simulink model "kundur_cvs_v3"  (R2025b)
settings: Solver=ode23t  StartTime=0.0  StopTime=0.5  MaxStep=0.005  RelTol=1e-3
values from neighbouring files (symbols this model uses):
  CCS_Load_amp_bus7 = 0    [kundur_cvs_v3_discrete_runtime.mat]    (also in kundur_cvs_v3_runtime.mat)
  CCS_Load_amp_bus9 = 0    [kundur_cvs_v3_discrete_runtime.mat]    (also in kundur_cvs_v3_runtime.mat)
  delta0_1 = 0.294539737007    [kundur_cvs_v3_discrete_runtime.mat]    (also in kundur_cvs_v3_runtime.mat)
  delta0_2 = 0.0944024626245    [kundur_cvs_v3_discrete_runtime.mat]    (also in kundur_cvs_v3_runtime.mat)
  delta0_3 = 0.25103283995    [kundur_cvs_v3_discrete_runtime.mat]    (also in kundur_cvs_v3_runtime.mat)
  delta0_4 = 0.0812572055811    [kundur_cvs_v3_discrete_runtime.mat]    (also in kundur_cvs_v3_runtime.mat)
  deltaG0_1 = 0.522124293082    [kundur_cvs_v3_discrete_runtime.mat]    (also in kundur_cvs_v3_runtime.mat)
  deltaG0_2 = 0.476153951225    [kundur_cvs_v3_discrete_runtime.mat]    (also in kundur_cvs_v3_runtime.mat)
  deltaG0_3 = 0.293879837027    [kundur_cvs_v3_discrete_runtime.mat]    (also in kundur_cvs_v3_runtime.mat)
  Dg_1 = 5    [kundur_cvs_v3_discrete_runtime.mat]    (also in kundur_cvs_v3_runtime.mat)
  Dg_2 = 5    [kundur_cvs_v3_discrete_runtime.mat]    (also in kundur_cvs_v3_runtime.mat)
  Dg_3 = 5    [kundur_cvs_v3_discrete_runtime.mat]    (also in kundur_cvs_v3_runtime.mat)
  LoadStep_amp_bus14 = 248000000    [kundur_cvs_v3_discrete_runtime.mat]    (also in kundur_cvs_v3_runtime.mat)
  LoadStep_amp_bus15 = 0    [kundur_cvs_v3_discrete_runtime.mat]    (also in kundur_cvs_v3_runtime.mat)
  LoadStep_trip_amp_bus14 = 0    [kundur_cvs_v3_discrete_runtime.mat]    (also in kundur_cvs_v3_runtime.mat)
  LoadStep_trip_amp_bus15 = 0    [kundur_cvs_v3_discrete_runtime.mat]    (also in kundur_cvs_v3_runtime.mat)
  Mg_1 = 13    [kundur_cvs_v3_discrete_runtime.mat]    (also in kundur_cvs_v3_runtime.mat)
  Mg_2 = 13    [kundur_cvs_v3_discrete_runtime.mat]    (also in kundur_cvs_v3_runtime.mat)
  Mg_3 = 12.35    [kundur_cvs_v3_discrete_runtime.mat]    (also in kundur_cvs_v3_runtime.mat)
  Pe_scale = 1e-08    [kundur_cvs_runtime.mat]    (also in kundur_cvs_v3_discrete_runtime.mat; kundur_cvs_v3_runtime.mat)
  Pm_1 = 0.250224865012    [kundur_cvs_v3_discrete_runtime.mat]    (also in kundur_cvs_v3_runtime.mat)
  Pm_2 = 0.250224865012    [kundur_cvs_v3_discrete_runtime.mat]    (also in kundur_cvs_v3_runtime.mat)
  Pm_3 = 0.250224865012    [kundur_cvs_v3_discrete_runtime.mat]    (also in kundur_cvs_v3_runtime.mat)
  Pm_4 = 0.250224865012    [kundur_cvs_v3_discrete_runtime.mat]    (also in kundur_cvs_v3_runtime.mat)
  Pmg_1 = 7.00000000011    [kundur_cvs_v3_discrete_runtime.mat]    (also in kundur_cvs_v3_runtime.mat)
  Pmg_2 = 7    [kundur_cvs_v3_discrete_runtime.mat]    (also in kundur_cvs_v3_runtime.mat)
  Pmg_3 = 7.19    [kundur_cvs_v3_discrete_runtime.mat]    (also in kundur_cvs_v3_runtime.mat)
  PmgStep_amp_1 = 0    [kundur_cvs_v3_discrete_runtime.mat]    (also in kundur_cvs_v3_runtime.mat)
  PmgStep_amp_2 = 0    [kundur_cvs_v3_discrete_runtime.mat]    (also in kundur_cvs_v3_runtime.mat)
  PmgStep_amp_3 = 0    [kundur_cvs_v3_discrete_runtime.mat]    (also in kundur_cvs_v3_runtime.mat)
  PmgStep_t_1 = 5    [kundur_cvs_v3_discrete_runtime.mat]    (also in kundur_cvs_v3_runtime.mat)
  PmgStep_t_2 = 5    [kundur_cvs_v3_discrete_runtime.mat]    (also in kundur_cvs_v3_runtime.mat)
  PmgStep_t_3 = 5    [kundur_cvs_v3_discrete_runtime.mat]    (also in kundur_cvs_v3_runtime.mat)
  Rg_1 = 0.05    [kundur_cvs_v3_discrete_runtime.mat]    (also in kundur_cvs_v3_runtime.mat)
  Rg_2 = 0.05    [kundur_cvs_v3_discrete_runtime.mat]    (also in kundur_cvs_v3_runtime.mat)
  Rg_3 = 0.05    [kundur_cvs_v3_discrete_runtime.mat]    (also in kundur_cvs_v3_runtime.mat)
  SGScale_1 = 0.111111111111    [kundur_cvs_v3_discrete_runtime.mat]    (also in kundur_cvs_v3_runtime.mat)
  SGScale_2 = 0.111111111111    [kundur_cvs_v3_discrete_runtime.mat]    (also in kundur_cvs_v3_runtime.mat)
  SGScale_3 = 0.111111111111    [kundur_cvs_v3_discrete_runtime.mat]    (also in kundur_cvs_v3_runtime.mat)
  Vbase_const = 230000    [kundur_cvs_runtime.mat]    (also in kundur_cvs_v3_discrete_runtime.mat; kundur_cvs_v3_runtime.mat)
  VemfG_1 = 266775.927939    [kundur_cvs_v3_discrete_runtime.mat]    (also in kundur_cvs_v3_runtime.mat)
  VemfG_2 = 255963.649879    [kundur_cvs_v3_discrete_runtime.mat]    (also in kundur_cvs_v3_runtime.mat)
  VemfG_3 = 266432.593136    [kundur_cvs_v3_discrete_runtime.mat]    (also in kundur_cvs_v3_runtime.mat)
  Vmag_1 = 230000    [kundur_cvs_runtime.mat]    (also in kundur_cvs_v3_discrete_runtime.mat = 201813.659575; kundur_cvs_v3_runtime.mat = 201813.659575)
  Vmag_2 = 230000    [kundur_cvs_runtime.mat]    (also in kundur_cvs_v3_discrete_runtime.mat = 232642.850172; kundur_cvs_v3_runtime.mat = 232642.850172)
  Vmag_3 = 230000    [kundur_cvs_runtime.mat]    (also in kundur_cvs_v3_discrete_runtime.mat = 178957.562058; kundur_cvs_v3_runtime.mat = 178957.562058)
  Vmag_4 = 230000    [kundur_cvs_runtime.mat]    (also in kundur_cvs_v3_discrete_runtime.mat = 226974.072481; kundur_cvs_v3_runtime.mat = 226974.072481)
  VSGScale_1 = 0.5    [kundur_cvs_v3_discrete_runtime.mat]    (also in kundur_cvs_v3_runtime.mat)
  VSGScale_2 = 0.5    [kundur_cvs_v3_discrete_runtime.mat]    (also in kundur_cvs_v3_runtime.mat)
  VSGScale_3 = 0.5    [kundur_cvs_v3_discrete_runtime.mat]    (also in kundur_cvs_v3_runtime.mat)
  VSGScale_4 = 0.5    [kundur_cvs_v3_discrete_runtime.mat]    (also in kundur_cvs_v3_runtime.mat)
  WindAmp_1 = 1    [kundur_cvs_v3_discrete_runtime.mat]    (also in kundur_cvs_v3_runtime.mat)
  WindAmp_2 = 1    [kundur_cvs_v3_discrete_runtime.mat]    (also in kundur_cvs_v3_runtime.mat)
  wn_const = 314.159265359    [kundur_cvs_runtime.mat]    (also in kundur_cvs_v3_discrete_runtime.mat; kundur_cvs_v3_runtime.mat)
  Wphase_1 = 0.0648179941055    [kundur_cvs_v3_discrete_runtime.mat]    (also in kundur_cvs_v3_runtime.mat)
  Wphase_2 = 0.0587091014116    [kundur_cvs_v3_discrete_runtime.mat]    (also in kundur_cvs_v3_runtime.mat)
  WVmag_1 = 230000    [kundur_cvs_v3_discrete_runtime.mat]    (also in kundur_cvs_v3_runtime.mat)
  WVmag_2 = 230000    [kundur_cvs_v3_discrete_runtime.mat]    (also in kundur_cvs_v3_runtime.mat)
undefined symbols (not defined in the file or in its folder): D_1, D_2, D_3, D_4, M_1, M_2, M_3, M_4, Pm_step_amp_1, Pm_step_amp_2, Pm_step_amp_3, Pm_step_amp_4, Pm_step_t_1, Pm_step_t_2, Pm_step_t_3, Pm_step_t_4
libraries: spsSeriesRLCBranchLib x72, spsGroundLib x57, spsControlledVoltageSourceLib x7, spsCurrentMeasurementLib x7, spsVoltageMeasurementLib x7, spsControlledCurrentSourceLib x4, spsACVoltageSourceLib x2, spspowerguiLib x1
settings Model: Creator=27443  LastModifiedBy=27443

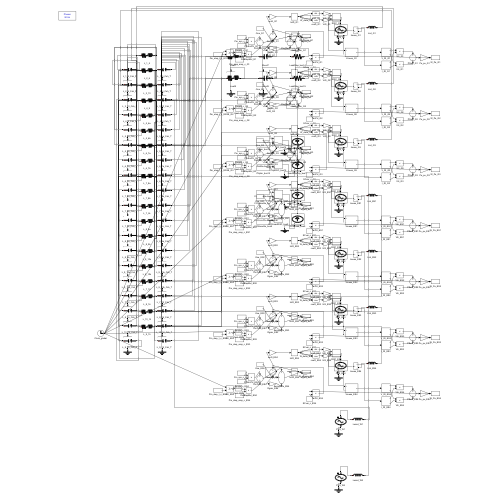
[thumbnail: Simulink's stored preview of the top-level diagram]
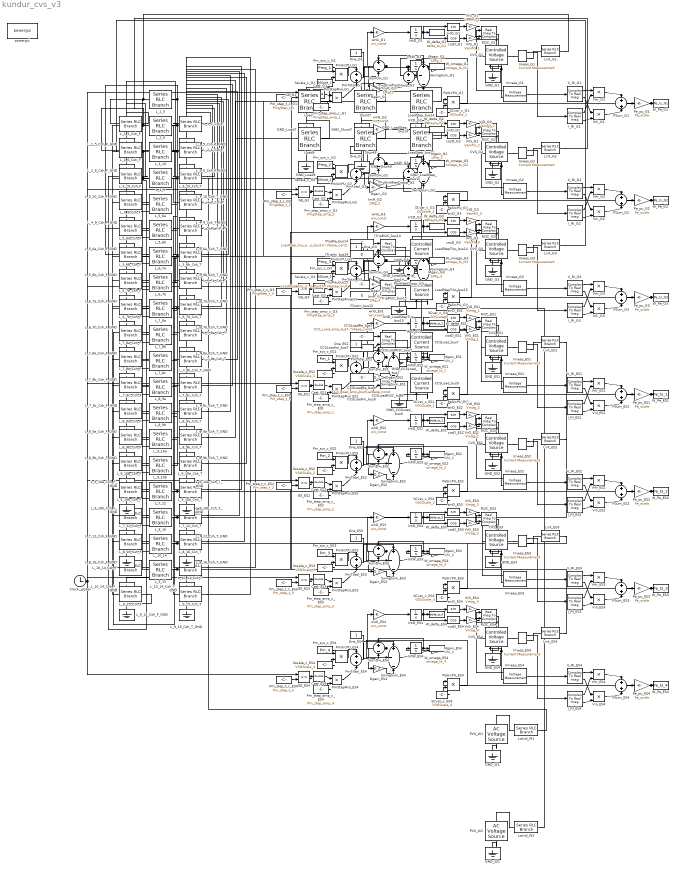
== system kundur_cvs_v3 ==
  CCSLoadIm_bus7 : Constant  Value=0
  CCSLoadIm_bus9 : Constant  Value=0
  CCSLoadRI2C_bus7 : RealImagToComplex
  CCSLoadRI2C_bus9 : RealImagToComplex
  CCSLoadRe_bus7 : Constant  Value=CCS_Load_amp_bus7 / Vbase_const
  CCSLoadRe_bus9 : Constant  Value=CCS_Load_amp_bus9 / Vbase_const
  CCSLoad_bus7 : spsControlledCurrentSourceLib/Controlled Current Source  Initialize=off  Source_Type=AC  Amplitude=0  Phase=0  Frequency=0  Measurements=None
  CCSLoad_bus9 : spsControlledCurrentSourceLib/Controlled Current Source  Initialize=off  Source_Type=AC  Amplitude=0  Phase=0  Frequency=0  Measurements=None
  CVS_ES1 : spsControlledVoltageSourceLib/Controlled Voltage Source  Initialize=off  Source_Type=DC  Amplitude=Vmag_1  Phase=0  Frequency=0  Measurements=None
  CVS_ES2 : spsControlledVoltageSourceLib/Controlled Voltage Source  Initialize=off  Source_Type=DC  Amplitude=Vmag_2  Phase=0  Frequency=0  Measurements=None
  CVS_ES3 : spsControlledVoltageSourceLib/Controlled Voltage Source  Initialize=off  Source_Type=DC  Amplitude=Vmag_3  Phase=0  Frequency=0  Measurements=None
  CVS_ES4 : spsControlledVoltageSourceLib/Controlled Voltage Source  Initialize=off  Source_Type=DC  Amplitude=Vmag_4  Phase=0  Frequency=0  Measurements=None
  CVS_G1 : spsControlledVoltageSourceLib/Controlled Voltage Source  Initialize=off  Source_Type=DC  Amplitude=VemfG_1  Phase=0  Frequency=0  Measurements=None
  CVS_G2 : spsControlledVoltageSourceLib/Controlled Voltage Source  Initialize=off  Source_Type=DC  Amplitude=VemfG_2  Phase=0  Frequency=0  Measurements=None
  CVS_G3 : spsControlledVoltageSourceLib/Controlled Voltage Source  Initialize=off  Source_Type=DC  Amplitude=VemfG_3  Phase=0  Frequency=0  Measurements=None
  Cast_ES{1..4} (4 alike) : DataTypeConversion  OutDataTypeStr=double  SaturateOnIntegerOverflow=off  RndMeth=Floor
  Cast_G1 : DataTypeConversion  OutDataTypeStr=double  SaturateOnIntegerOverflow=off  RndMeth=Floor
  Cast_G2 : DataTypeConversion  OutDataTypeStr=double  SaturateOnIntegerOverflow=off  RndMeth=Floor
  Cast_G3 : DataTypeConversion  OutDataTypeStr=double  SaturateOnIntegerOverflow=off  RndMeth=Floor
  Clock_global : Clock
  Dgain_ES1 : Gain  Gain=D_1
  Dgain_ES2 : Gain  Gain=D_2
  Dgain_ES3 : Gain  Gain=D_3
  Dgain_ES4 : Gain  Gain=D_4
  Dgain_G1 : Gain  Gain=Dg_1
  Dgain_G2 : Gain  Gain=Dg_2
  Dgain_G3 : Gain  Gain=Dg_3
  GE_ES{1..4} (4 alike) : RelationalOperator  OutDataTypeStr=boolean  RndMeth=Simplest  InputSameDT=off
  GE_G1 : RelationalOperator  OutDataTypeStr=boolean  RndMeth=Simplest  InputSameDT=off
  GE_G2 : RelationalOperator  OutDataTypeStr=boolean  RndMeth=Simplest  InputSameDT=off
  GE_G3 : RelationalOperator  OutDataTypeStr=boolean  RndMeth=Simplest  InputSameDT=off
  GND_CCSLoad_bus7 : spsGroundLib/Ground  LConnTagsString=a
  GND_CCSLoad_bus9 : spsGroundLib/Ground  LConnTagsString=a
  GND_ES{1..4} (4 alike) : spsGroundLib/Ground  LConnTagsString=a
  GND_G1 : spsGroundLib/Ground  LConnTagsString=a
  GND_G2 : spsGroundLib/Ground  LConnTagsString=a
  GND_G3 : spsGroundLib/Ground  LConnTagsString=a
  GND_Load7 : spsGroundLib/Ground  LConnTagsString=a
  GND_Load9 : spsGroundLib/Ground  LConnTagsString=a
  GND_LoadStepTrip_bus14 : spsGroundLib/Ground  LConnTagsString=a
  GND_LoadStepTrip_bus15 : spsGroundLib/Ground  LConnTagsString=a
  GND_LoadStep_bus14 : spsGroundLib/Ground  LConnTagsString=a
  GND_LoadStep_bus15 : spsGroundLib/Ground  LConnTagsString=a
  GND_Shunt7 : spsGroundLib/Ground  LConnTagsString=a
  GND_Shunt9 : spsGroundLib/Ground  LConnTagsString=a
  GND_W1 : spsGroundLib/Ground  LConnTagsString=a
  GND_W2 : spsGroundLib/Ground  LConnTagsString=a
  ITripIm_bus14 : Constant  Value=0
  ITripIm_bus15 : Constant  Value=0
  ITripRI2C_bus14 : RealImagToComplex
  ITripRI2C_bus15 : RealImagToComplex
  ITripRe_bus14 : Constant  Value=LoadStep_trip_amp_bus14 / Vbase_const
  ITripRe_bus15 : Constant  Value=LoadStep_trip_amp_bus15 / Vbase_const
  I_RI_ES{1..4} (4 alike) : ComplexToRealImag
  I_RI_G1 : ComplexToRealImag
  I_RI_G2 : ComplexToRealImag
  I_RI_G3 : ComplexToRealImag
  Imeas_ES{1..4} (4 alike) : spsCurrentMeasurementLib/Current Measurement  PhasorSimulation=on  OutputType=Complex  PSBequivalent=0
  Imeas_G1 : spsCurrentMeasurementLib/Current Measurement  PhasorSimulation=on  OutputType=Complex  PSBequivalent=0
  Imeas_G2 : spsCurrentMeasurementLib/Current Measurement  PhasorSimulation=on  OutputType=Complex  PSBequivalent=0
  Imeas_G3 : spsCurrentMeasurementLib/Current Measurement  PhasorSimulation=on  OutputType=Complex  PSBequivalent=0
  IntD_ES1 : Integrator  InitialCondition=delta0_1
  IntD_ES2 : Integrator  InitialCondition=delta0_2
  IntD_ES3 : Integrator  InitialCondition=delta0_3
  IntD_ES4 : Integrator  InitialCondition=delta0_4
  IntD_G1 : Integrator  InitialCondition=deltaG0_1
  IntD_G2 : Integrator  InitialCondition=deltaG0_2
  IntD_G3 : Integrator  InitialCondition=deltaG0_3
  IntW_ES{1..4} (4 alike) : Integrator  InitialCondition=1
  IntW_G1 : Integrator  InitialCondition=1
  IntW_G2 : Integrator  InitialCondition=1
  IntW_G3 : Integrator  InitialCondition=1
  InvR_G1 : Gain  Gain=1/Rg_1
  InvR_G2 : Gain  Gain=1/Rg_2
  InvR_G3 : Gain  Gain=1/Rg_3
  L_10_14 : spsSeriesRLCBranchLib/Series RLC Branch  LConnTagsString=__new0  RConnTagsString=__new0  BranchType=RL  Resistance=0.01  Inductance=0.0005  SetiL0=off  InitialCurrent=0  Capacitance=1e-6  Setx0=off  InitialVoltage=0  Measurements=None
  L_10_14_Csh_F : spsSeriesRLCBranchLib/Series RLC Branch  LConnTagsString=__new0  RConnTagsString=__new0  BranchType=C  Resistance=1  Inductance=1e-3  SetiL0=off  InitialCurrent=0  Capacitance=4.5e-09  Setx0=off  InitialVoltage=0  Measurements=None
  L_10_14_Csh_F_GND : spsGroundLib/Ground  LConnTagsString=a
  L_10_14_Csh_T : spsSeriesRLCBranchLib/Series RLC Branch  LConnTagsString=__new0  RConnTagsString=__new0  BranchType=C  Resistance=1  Inductance=1e-3  SetiL0=off  InitialCurrent=0  Capacitance=4.5e-09  Setx0=off  InitialVoltage=0  Measurements=None
  L_10_14_Csh_T_GND : spsGroundLib/Ground  LConnTagsString=a
  L_1_5 : spsSeriesRLCBranchLib/Series RLC Branch  LConnTagsString=__new0  RConnTagsString=__new0  BranchType=RL  Resistance=0.265  Inductance=0.00705  SetiL0=off  InitialCurrent=0  Capacitance=1e-6  Setx0=off  InitialVoltage=0  Measurements=None
  L_1_5_Csh_F : spsSeriesRLCBranchLib/Series RLC Branch  LConnTagsString=__new0  RConnTagsString=__new0  BranchType=C  Resistance=1  Inductance=1e-3  SetiL0=off  InitialCurrent=0  Capacitance=2.25e-08  Setx0=off  InitialVoltage=0  Measurements=None
  L_1_5_Csh_F_GND : spsGroundLib/Ground  LConnTagsString=a
  L_1_5_Csh_T : spsSeriesRLCBranchLib/Series RLC Branch  LConnTagsString=__new0  RConnTagsString=__new0  BranchType=C  Resistance=1  Inductance=1e-3  SetiL0=off  InitialCurrent=0  Capacitance=2.25e-08  Setx0=off  InitialVoltage=0  Measurements=None
  L_1_5_Csh_T_GND : spsGroundLib/Ground  LConnTagsString=a
  L_2_6 : spsSeriesRLCBranchLib/Series RLC Branch  LConnTagsString=__new0  RConnTagsString=__new0  BranchType=RL  Resistance=0.265  Inductance=0.00705  SetiL0=off  InitialCurrent=0  Capacitance=1e-6  Setx0=off  InitialVoltage=0  Measurements=None
  L_2_6_Csh_F : spsSeriesRLCBranchLib/Series RLC Branch  LConnTagsString=__new0  RConnTagsString=__new0  BranchType=C  Resistance=1  Inductance=1e-3  SetiL0=off  InitialCurrent=0  Capacitance=2.25e-08  Setx0=off  InitialVoltage=0  Measurements=None
  L_2_6_Csh_F_GND : spsGroundLib/Ground  LConnTagsString=a
  L_2_6_Csh_T : spsSeriesRLCBranchLib/Series RLC Branch  LConnTagsString=__new0  RConnTagsString=__new0  BranchType=C  Resistance=1  Inductance=1e-3  SetiL0=off  InitialCurrent=0  Capacitance=2.25e-08  Setx0=off  InitialVoltage=0  Measurements=None
  L_2_6_Csh_T_GND : spsGroundLib/Ground  LConnTagsString=a
  L_3_10 : spsSeriesRLCBranchLib/Series RLC Branch  LConnTagsString=__new0  RConnTagsString=__new0  BranchType=RL  Resistance=0.265  Inductance=0.00705  SetiL0=off  InitialCurrent=0  Capacitance=1e-6  Setx0=off  InitialVoltage=0  Measurements=None
  L_3_10_Csh_F : spsSeriesRLCBranchLib/Series RLC Branch  LConnTagsString=__new0  RConnTagsString=__new0  BranchType=C  Resistance=1  Inductance=1e-3  SetiL0=off  InitialCurrent=0  Capacitance=2.25e-08  Setx0=off  InitialVoltage=0  Measurements=None
  L_3_10_Csh_F_GND : spsGroundLib/Ground  LConnTagsString=a
  L_3_10_Csh_T : spsSeriesRLCBranchLib/Series RLC Branch  LConnTagsString=__new0  RConnTagsString=__new0  BranchType=C  Resistance=1  Inductance=1e-3  SetiL0=off  InitialCurrent=0  Capacitance=2.25e-08  Setx0=off  InitialVoltage=0  Measurements=None
  L_3_10_Csh_T_GND : spsGroundLib/Ground  LConnTagsString=a
  L_4_9 : spsSeriesRLCBranchLib/Series RLC Branch  LConnTagsString=__new0  RConnTagsString=__new0  BranchType=RL  Resistance=0.265  Inductance=0.00705  SetiL0=off  InitialCurrent=0  Capacitance=1e-6  Setx0=off  InitialVoltage=0  Measurements=None
  L_4_9_Csh_F : spsSeriesRLCBranchLib/Series RLC Branch  LConnTagsString=__new0  RConnTagsString=__new0  BranchType=C  Resistance=1  Inductance=1e-3  SetiL0=off  InitialCurrent=0  Capacitance=2.25e-08  Setx0=off  InitialVoltage=0  Measurements=None
  L_4_9_Csh_F_GND : spsGroundLib/Ground  LConnTagsString=a
  L_4_9_Csh_T : spsSeriesRLCBranchLib/Series RLC Branch  LConnTagsString=__new0  RConnTagsString=__new0  BranchType=C  Resistance=1  Inductance=1e-3  SetiL0=off  InitialCurrent=0  Capacitance=2.25e-08  Setx0=off  InitialVoltage=0  Measurements=None
  L_4_9_Csh_T_GND : spsGroundLib/Ground  LConnTagsString=a
  L_5_6a : spsSeriesRLCBranchLib/Series RLC Branch  LConnTagsString=__new0  RConnTagsString=__new0  BranchType=RL  Resistance=1.325  Inductance=0.03525  SetiL0=off  InitialCurrent=0  Capacitance=1e-6  Setx0=off  InitialVoltage=0  Measurements=None
  L_5_6a_Csh_F : spsSeriesRLCBranchLib/Series RLC Branch  LConnTagsString=__new0  RConnTagsString=__new0  BranchType=C  Resistance=1  Inductance=1e-3  SetiL0=off  InitialCurrent=0  Capacitance=1.125e-07  Setx0=off  InitialVoltage=0  Measurements=None
  L_5_6a_Csh_F_GND : spsGroundLib/Ground  LConnTagsString=a
  L_5_6a_Csh_T : spsSeriesRLCBranchLib/Series RLC Branch  LConnTagsString=__new0  RConnTagsString=__new0  BranchType=C  Resistance=1  Inductance=1e-3  SetiL0=off  InitialCurrent=0  Capacitance=1.125e-07  Setx0=off  InitialVoltage=0  Measurements=None
  L_5_6a_Csh_T_GND : spsGroundLib/Ground  LConnTagsString=a
  L_5_6b : spsSeriesRLCBranchLib/Series RLC Branch  LConnTagsString=__new0  RConnTagsString=__new0  BranchType=RL  Resistance=1.325  Inductance=0.03525  SetiL0=off  InitialCurrent=0  Capacitance=1e-6  Setx0=off  InitialVoltage=0  Measurements=None
  L_5_6b_Csh_F : spsSeriesRLCBranchLib/Series RLC Branch  LConnTagsString=__new0  RConnTagsString=__new0  BranchType=C  Resistance=1  Inductance=1e-3  SetiL0=off  InitialCurrent=0  Capacitance=1.125e-07  Setx0=off  InitialVoltage=0  Measurements=None
  L_5_6b_Csh_F_GND : spsGroundLib/Ground  LConnTagsString=a
  L_5_6b_Csh_T : spsSeriesRLCBranchLib/Series RLC Branch  LConnTagsString=__new0  RConnTagsString=__new0  BranchType=C  Resistance=1  Inductance=1e-3  SetiL0=off  InitialCurrent=0  Capacitance=1.125e-07  Setx0=off  InitialVoltage=0  Measurements=None
  L_5_6b_Csh_T_GND : spsGroundLib/Ground  LConnTagsString=a
  L_6_7a : spsSeriesRLCBranchLib/Series RLC Branch  LConnTagsString=__new0  RConnTagsString=__new0  BranchType=RL  Resistance=0.53  Inductance=0.0141  SetiL0=off  InitialCurrent=0  Capacitance=1e-6  Setx0=off  InitialVoltage=0  Measurements=None
  L_6_7a_Csh_F : spsSeriesRLCBranchLib/Series RLC Branch  LConnTagsString=__new0  RConnTagsString=__new0  BranchType=C  Resistance=1  Inductance=1e-3  SetiL0=off  InitialCurrent=0  Capacitance=4.5e-08  Setx0=off  InitialVoltage=0  Measurements=None
  L_6_7a_Csh_F_GND : spsGroundLib/Ground  LConnTagsString=a
  L_6_7a_Csh_T : spsSeriesRLCBranchLib/Series RLC Branch  LConnTagsString=__new0  RConnTagsString=__new0  BranchType=C  Resistance=1  Inductance=1e-3  SetiL0=off  InitialCurrent=0  Capacitance=4.5e-08  Setx0=off  InitialVoltage=0  Measurements=None
  L_6_7a_Csh_T_GND : spsGroundLib/Ground  LConnTagsString=a
  L_6_7b : spsSeriesRLCBranchLib/Series RLC Branch  LConnTagsString=__new0  RConnTagsString=__new0  BranchType=RL  Resistance=0.53  Inductance=0.0141  SetiL0=off  InitialCurrent=0  Capacitance=1e-6  Setx0=off  InitialVoltage=0  Measurements=None
  L_6_7b_Csh_F : spsSeriesRLCBranchLib/Series RLC Branch  LConnTagsString=__new0  RConnTagsString=__new0  BranchType=C  Resistance=1  Inductance=1e-3  SetiL0=off  InitialCurrent=0  Capacitance=4.5e-08  Setx0=off  InitialVoltage=0  Measurements=None
  L_6_7b_Csh_F_GND : spsGroundLib/Ground  LConnTagsString=a
  L_6_7b_Csh_T : spsSeriesRLCBranchLib/Series RLC Branch  LConnTagsString=__new0  RConnTagsString=__new0  BranchType=C  Resistance=1  Inductance=1e-3  SetiL0=off  InitialCurrent=0  Capacitance=4.5e-08  Setx0=off  InitialVoltage=0  Measurements=None
  L_6_7b_Csh_T_GND : spsGroundLib/Ground  LConnTagsString=a
  L_7_12 : spsSeriesRLCBranchLib/Series RLC Branch  LConnTagsString=__new0  RConnTagsString=__new0  BranchType=RL  Resistance=0.01  Inductance=0.0005  SetiL0=off  InitialCurrent=0  Capacitance=1e-6  Setx0=off  InitialVoltage=0  Measurements=None
  L_7_12_Csh_F : spsSeriesRLCBranchLib/Series RLC Branch  LConnTagsString=__new0  RConnTagsString=__new0  BranchType=C  Resistance=1  Inductance=1e-3  SetiL0=off  InitialCurrent=0  Capacitance=4.5e-09  Setx0=off  InitialVoltage=0  Measurements=None
  L_7_12_Csh_F_GND : spsGroundLib/Ground  LConnTagsString=a
  L_7_12_Csh_T : spsSeriesRLCBranchLib/Series RLC Branch  LConnTagsString=__new0  RConnTagsString=__new0  BranchType=C  Resistance=1  Inductance=1e-3  SetiL0=off  InitialCurrent=0  Capacitance=4.5e-09  Setx0=off  InitialVoltage=0  Measurements=None
  L_7_12_Csh_T_GND : spsGroundLib/Ground  LConnTagsString=a
  L_7_8a : spsSeriesRLCBranchLib/Series RLC Branch  LConnTagsString=__new0  RConnTagsString=__new0  BranchType=RL  Resistance=5.83  Inductance=0.1551  SetiL0=off  InitialCurrent=0  Capacitance=1e-6  Setx0=off  InitialVoltage=0  Measurements=None
  L_7_8a_Csh_F : spsSeriesRLCBranchLib/Series RLC Branch  LConnTagsString=__new0  RConnTagsString=__new0  BranchType=C  Resistance=1  Inductance=1e-3  SetiL0=off  InitialCurrent=0  Capacitance=4.95e-07  Setx0=off  InitialVoltage=0  Measurements=None
  L_7_8a_Csh_F_GND : spsGroundLib/Ground  LConnTagsString=a
  L_7_8a_Csh_T : spsSeriesRLCBranchLib/Series RLC Branch  LConnTagsString=__new0  RConnTagsString=__new0  BranchType=C  Resistance=1  Inductance=1e-3  SetiL0=off  InitialCurrent=0  Capacitance=4.95e-07  Setx0=off  InitialVoltage=0  Measurements=None
  L_7_8a_Csh_T_GND : spsGroundLib/Ground  LConnTagsString=a
  L_7_8b : spsSeriesRLCBranchLib/Series RLC Branch  LConnTagsString=__new0  RConnTagsString=__new0  BranchType=RL  Resistance=5.83  Inductance=0.1551  SetiL0=off  InitialCurrent=0  Capacitance=1e-6  Setx0=off  InitialVoltage=0  Measurements=None
  L_7_8b_Csh_F : spsSeriesRLCBranchLib/Series RLC Branch  LConnTagsString=__new0  RConnTagsString=__new0  BranchType=C  Resistance=1  Inductance=1e-3  SetiL0=off  InitialCurrent=0  Capacitance=4.95e-07  Setx0=off  InitialVoltage=0  Measurements=None
  L_7_8b_Csh_F_GND : spsGroundLib/Ground  LConnTagsString=a
  L_7_8b_Csh_T : spsSeriesRLCBranchLib/Series RLC Branch  LConnTagsString=__new0  RConnTagsString=__new0  BranchType=C  Resistance=1  Inductance=1e-3  SetiL0=off  InitialCurrent=0  Capacitance=4.95e-07  Setx0=off  InitialVoltage=0  Measurements=None
  L_7_8b_Csh_T_GND : spsGroundLib/Ground  LConnTagsString=a
  L_7_8c : spsSeriesRLCBranchLib/Series RLC Branch  LConnTagsString=__new0  RConnTagsString=__new0  BranchType=RL  Resistance=5.83  Inductance=0.1551  SetiL0=off  InitialCurrent=0  Capacitance=1e-6  Setx0=off  InitialVoltage=0  Measurements=None
  L_7_8c_Csh_F : spsSeriesRLCBranchLib/Series RLC Branch  LConnTagsString=__new0  RConnTagsString=__new0  BranchType=C  Resistance=1  Inductance=1e-3  SetiL0=off  InitialCurrent=0  Capacitance=4.95e-07  Setx0=off  InitialVoltage=0  Measurements=None
  L_7_8c_Csh_F_GND : spsGroundLib/Ground  LConnTagsString=a
  L_7_8c_Csh_T : spsSeriesRLCBranchLib/Series RLC Branch  LConnTagsString=__new0  RConnTagsString=__new0  BranchType=C  Resistance=1  Inductance=1e-3  SetiL0=off  InitialCurrent=0  Capacitance=4.95e-07  Setx0=off  InitialVoltage=0  Measurements=None
  L_7_8c_Csh_T_GND : spsGroundLib/Ground  LConnTagsString=a
  L_8_16 : spsSeriesRLCBranchLib/Series RLC Branch  LConnTagsString=__new0  RConnTagsString=__new0  BranchType=RL  Resistance=0.01  Inductance=0.0005  SetiL0=off  InitialCurrent=0  Capacitance=1e-6  Setx0=off  InitialVoltage=0  Measurements=None
  L_8_16_Csh_F : spsSeriesRLCBranchLib/Series RLC Branch  LConnTagsString=__new0  RConnTagsString=__new0  BranchType=C  Resistance=1  Inductance=1e-3  SetiL0=off  InitialCurrent=0  Capacitance=4.5e-09  Setx0=off  InitialVoltage=0  Measurements=None
  L_8_16_Csh_F_GND : spsGroundLib/Ground  LConnTagsString=a
  L_8_16_Csh_T : spsSeriesRLCBranchLib/Series RLC Branch  LConnTagsString=__new0  RConnTagsString=__new0  BranchType=C  Resistance=1  Inductance=1e-3  SetiL0=off  InitialCurrent=0  Capacitance=4.5e-09  Setx0=off  InitialVoltage=0  Measurements=None
  L_8_16_Csh_T_GND : spsGroundLib/Ground  LConnTagsString=a
  L_8_9a : spsSeriesRLCBranchLib/Series RLC Branch  LConnTagsString=__new0  RConnTagsString=__new0  BranchType=RL  Resistance=0.53  Inductance=0.0141  SetiL0=off  InitialCurrent=0  Capacitance=1e-6  Setx0=off  InitialVoltage=0  Measurements=None
  L_8_9a_Csh_F : spsSeriesRLCBranchLib/Series RLC Branch  LConnTagsString=__new0  RConnTagsString=__new0  BranchType=C  Resistance=1  Inductance=1e-3  SetiL0=off  InitialCurrent=0  Capacitance=4.5e-08  Setx0=off  InitialVoltage=0  Measurements=None
  L_8_9a_Csh_F_GND : spsGroundLib/Ground  LConnTagsString=a
  L_8_9a_Csh_T : spsSeriesRLCBranchLib/Series RLC Branch  LConnTagsString=__new0  RConnTagsString=__new0  BranchType=C  Resistance=1  Inductance=1e-3  SetiL0=off  InitialCurrent=0  Capacitance=4.5e-08  Setx0=off  InitialVoltage=0  Measurements=None
  L_8_9a_Csh_T_GND : spsGroundLib/Ground  LConnTagsString=a
  L_8_9b : spsSeriesRLCBranchLib/Series RLC Branch  LConnTagsString=__new0  RConnTagsString=__new0  BranchType=RL  Resistance=0.53  Inductance=0.0141  SetiL0=off  InitialCurrent=0  Capacitance=1e-6  Setx0=off  InitialVoltage=0  Measurements=None
  L_8_9b_Csh_F : spsSeriesRLCBranchLib/Series RLC Branch  LConnTagsString=__new0  RConnTagsString=__new0  BranchType=C  Resistance=1  Inductance=1e-3  SetiL0=off  InitialCurrent=0  Capacitance=4.5e-08  Setx0=off  InitialVoltage=0  Measurements=None
  L_8_9b_Csh_F_GND : spsGroundLib/Ground  LConnTagsString=a
  L_8_9b_Csh_T : spsSeriesRLCBranchLib/Series RLC Branch  LConnTagsString=__new0  RConnTagsString=__new0  BranchType=C  Resistance=1  Inductance=1e-3  SetiL0=off  InitialCurrent=0  Capacitance=4.5e-08  Setx0=off  InitialVoltage=0  Measurements=None
  L_8_9b_Csh_T_GND : spsGroundLib/Ground  LConnTagsString=a
  L_9_10a : spsSeriesRLCBranchLib/Series RLC Branch  LConnTagsString=__new0  RConnTagsString=__new0  BranchType=RL  Resistance=1.325  Inductance=0.03525  SetiL0=off  InitialCurrent=0  Capacitance=1e-6  Setx0=off  InitialVoltage=0  Measurements=None
  L_9_10a_Csh_F : spsSeriesRLCBranchLib/Series RLC Branch  LConnTagsString=__new0  RConnTagsString=__new0  BranchType=C  Resistance=1  Inductance=1e-3  SetiL0=off  InitialCurrent=0  Capacitance=1.125e-07  Setx0=off  InitialVoltage=0  Measurements=None
  L_9_10a_Csh_F_GND : spsGroundLib/Ground  LConnTagsString=a
  L_9_10a_Csh_T : spsSeriesRLCBranchLib/Series RLC Branch  LConnTagsString=__new0  RConnTagsString=__new0  BranchType=C  Resistance=1  Inductance=1e-3  SetiL0=off  InitialCurrent=0  Capacitance=1.125e-07  Setx0=off  InitialVoltage=0  Measurements=None
  L_9_10a_Csh_T_GND : spsGroundLib/Ground  LConnTagsString=a
  L_9_10b : spsSeriesRLCBranchLib/Series RLC Branch  LConnTagsString=__new0  RConnTagsString=__new0  BranchType=RL  Resistance=1.325  Inductance=0.03525  SetiL0=off  InitialCurrent=0  Capacitance=1e-6  Setx0=off  InitialVoltage=0  Measurements=None
  L_9_10b_Csh_F : spsSeriesRLCBranchLib/Series RLC Branch  LConnTagsString=__new0  RConnTagsString=__new0  BranchType=C  Resistance=1  Inductance=1e-3  SetiL0=off  InitialCurrent=0  Capacitance=1.125e-07  Setx0=off  InitialVoltage=0  Measurements=None
  L_9_10b_Csh_F_GND : spsGroundLib/Ground  LConnTagsString=a
  L_9_10b_Csh_T : spsSeriesRLCBranchLib/Series RLC Branch  LConnTagsString=__new0  RConnTagsString=__new0  BranchType=C  Resistance=1  Inductance=1e-3  SetiL0=off  InitialCurrent=0  Capacitance=1.125e-07  Setx0=off  InitialVoltage=0  Measurements=None
  L_9_10b_Csh_T_GND : spsGroundLib/Ground  LConnTagsString=a
  L_9_15 : spsSeriesRLCBranchLib/Series RLC Branch  LConnTagsString=__new0  RConnTagsString=__new0  BranchType=RL  Resistance=0.01  Inductance=0.0005  SetiL0=off  InitialCurrent=0  Capacitance=1e-6  Setx0=off  InitialVoltage=0  Measurements=None
  L_9_15_Csh_F : spsSeriesRLCBranchLib/Series RLC Branch  LConnTagsString=__new0  RConnTagsString=__new0  BranchType=C  Resistance=1  Inductance=1e-3  SetiL0=off  InitialCurrent=0  Capacitance=4.5e-09  Setx0=off  InitialVoltage=0  Measurements=None
  L_9_15_Csh_F_GND : spsGroundLib/Ground  LConnTagsString=a
  L_9_15_Csh_T : spsSeriesRLCBranchLib/Series RLC Branch  LConnTagsString=__new0  RConnTagsString=__new0  BranchType=C  Resistance=1  Inductance=1e-3  SetiL0=off  InitialCurrent=0  Capacitance=4.5e-09  Setx0=off  InitialVoltage=0  Measurements=None
  L_9_15_Csh_T_GND : spsGroundLib/Ground  LConnTagsString=a
  Lint_ES{1..4} (4 alike) : spsSeriesRLCBranchLib/Series RLC Branch  LConnTagsString=__new0  RConnTagsString=__new0  BranchType=L  Resistance=1  Inductance=0.2525788947  SetiL0=off  InitialCurrent=0  Capacitance=1e-6  Setx0=off  InitialVoltage=0  Measurements=None
  Lint_G1 : spsSeriesRLCBranchLib/Series RLC Branch  LConnTagsString=__new0  RConnTagsString=__new0  BranchType=L  Resistance=1  Inductance=0.05612864326  SetiL0=off  InitialCurrent=0  Capacitance=1e-6  Setx0=off  InitialVoltage=0  Measurements=None
  Lint_G2 : spsSeriesRLCBranchLib/Series RLC Branch  LConnTagsString=__new0  RConnTagsString=__new0  BranchType=L  Resistance=1  Inductance=0.05612864326  SetiL0=off  InitialCurrent=0  Capacitance=1e-6  Setx0=off  InitialVoltage=0  Measurements=None
  Lint_G3 : spsSeriesRLCBranchLib/Series RLC Branch  LConnTagsString=__new0  RConnTagsString=__new0  BranchType=L  Resistance=1  Inductance=0.05612864326  SetiL0=off  InitialCurrent=0  Capacitance=1e-6  Setx0=off  InitialVoltage=0  Measurements=None
  Load7 : spsSeriesRLCBranchLib/Series RLC Branch  LConnTagsString=__new0  RConnTagsString=__new0  BranchType=RL  Resistance=54.70527404  Inductance=1.683859298  SetiL0=off  InitialCurrent=0  Capacitance=1e-6  Setx0=off  InitialVoltage=0  Measurements=None
  Load9 : spsSeriesRLCBranchLib/Series RLC Branch  LConnTagsString=__new0  RConnTagsString=__new0  BranchType=RL  Resistance=29.93774759  Inductance=1.683859298  SetiL0=off  InitialCurrent=0  Capacitance=1e-6  Setx0=off  InitialVoltage=0  Measurements=None
  LoadStepTrip_bus14 : spsControlledCurrentSourceLib/Controlled Current Source  Initialize=off  Source_Type=AC  Amplitude=0  Phase=0  Frequency=0  Measurements=None
  LoadStepTrip_bus15 : spsControlledCurrentSourceLib/Controlled Current Source  Initialize=off  Source_Type=AC  Amplitude=0  Phase=0  Frequency=0  Measurements=None
  LoadStep_bus14 : spsSeriesRLCBranchLib/Series RLC Branch  LConnTagsString=__new0  RConnTagsString=__new0  BranchType=R  Resistance=Vbase_const^2 / max(LoadStep_amp_bus14, 1e-3)  Inductance=1e-3  SetiL0=off  InitialCurrent=0  Capacitance=1e-6  Setx0=off  InitialVoltage=0  Measurements=None
  LoadStep_bus15 : spsSeriesRLCBranchLib/Series RLC Branch  LConnTagsString=__new0  RConnTagsString=__new0  BranchType=R  Resistance=Vbase_const^2 / max(LoadStep_amp_bus15, 1e-3)  Inductance=1e-3  SetiL0=off  InitialCurrent=0  Capacitance=1e-6  Setx0=off  InitialVoltage=0  Measurements=None
  Lwind_W1 : spsSeriesRLCBranchLib/Series RLC Branch  LConnTagsString=__new0  RConnTagsString=__new0  BranchType=L  Resistance=1  Inductance=1e-6  SetiL0=off  InitialCurrent=0  Capacitance=1e-6  Setx0=off  InitialVoltage=0  Measurements=None
  Lwind_W2 : spsSeriesRLCBranchLib/Series RLC Branch  LConnTagsString=__new0  RConnTagsString=__new0  BranchType=L  Resistance=1  Inductance=1e-6  SetiL0=off  InitialCurrent=0  Capacitance=1e-6  Setx0=off  InitialVoltage=0  Measurements=None
  Mgain_ES1 : Gain  Gain=1/M_1
  Mgain_ES2 : Gain  Gain=1/M_2
  Mgain_ES3 : Gain  Gain=1/M_3
  Mgain_ES4 : Gain  Gain=1/M_4
  Mgain_G1 : Gain  Gain=1/Mg_1
  Mgain_G2 : Gain  Gain=1/Mg_2
  Mgain_G3 : Gain  Gain=1/Mg_3
  One_ES{1..4} (4 alike) : Constant
  One_G1 : Constant
  One_G2 : Constant
  One_G3 : Constant
  PSum_ES{1..4} (4 alike) : Sum
  PSum_G1 : Sum
  PSum_G2 : Sum
  PSum_G3 : Sum
  PVS_W1 : spsACVoltageSourceLib/AC Voltage Source  Amplitude=(WindAmp_1) * (WVmag_1)  Phase=(Wphase_1) * 180/pi  Frequency=50  SampleTime=0  Measurements=None  BusType=swing  Pref=10e3  Qref=0  Qmin=-inf  Qmax=+inf
  PVS_W2 : spsACVoltageSourceLib/AC Voltage Source  Amplitude=(WindAmp_2) * (WVmag_2)  Phase=(Wphase_2) * 180/pi  Frequency=50  SampleTime=0  Measurements=None  BusType=swing  Pref=10e3  Qref=0  Qmin=-inf  Qmax=+inf
  PeSrcPU_ES{1..4} (4 alike) : Product
  PeSrcPU_G1 : Product
  PeSrcPU_G2 : Product
  PeSrcPU_G3 : Product
  Pe_pu_ES{1..4} (4 alike) : Gain  Gain=Pe_scale
  Pe_pu_G1 : Gain  Gain=Pe_scale
  Pe_pu_G2 : Gain  Gain=Pe_scale
  Pe_pu_G3 : Gain  Gain=Pe_scale
  PmAfterDroop_G1 : Sum  Inputs=+-
  PmAfterDroop_G2 : Sum  Inputs=+-
  PmAfterDroop_G3 : Sum  Inputs=+-
  PmSrcPU_ES{1..4} (4 alike) : Product
  PmSrcPU_G1 : Product
  PmSrcPU_G2 : Product
  PmSrcPU_G3 : Product
  PmStepMul_ES{1..4} (4 alike) : Product
  PmStepMul_G1 : Product
  PmStepMul_G2 : Product
  PmStepMul_G3 : Product
  PmTotal_ES{1..4} (4 alike) : Sum
  PmTotal_G1 : Sum
  PmTotal_G2 : Sum
  PmTotal_G3 : Sum
  Pm_step_amp_c_ES1 : Constant  Value=Pm_step_amp_1
  Pm_step_amp_c_ES2 : Constant  Value=Pm_step_amp_2
  Pm_step_amp_c_ES3 : Constant  Value=Pm_step_amp_3
  Pm_step_amp_c_ES4 : Constant  Value=Pm_step_amp_4
  Pm_step_amp_c_G1 : Constant  Value=PmgStep_amp_1
  Pm_step_amp_c_G2 : Constant  Value=PmgStep_amp_2
  Pm_step_amp_c_G3 : Constant  Value=PmgStep_amp_3
  Pm_step_t_c_ES1 : Constant  Value=Pm_step_t_1
  Pm_step_t_c_ES2 : Constant  Value=Pm_step_t_2
  Pm_step_t_c_ES3 : Constant  Value=Pm_step_t_3
  Pm_step_t_c_ES4 : Constant  Value=Pm_step_t_4
  Pm_step_t_c_G1 : Constant  Value=PmgStep_t_1
  Pm_step_t_c_G2 : Constant  Value=PmgStep_t_2
  Pm_step_t_c_G3 : Constant  Value=PmgStep_t_3
  Pm_sys_c_ES1 : Constant  Value=Pm_1
  Pm_sys_c_ES2 : Constant  Value=Pm_2
  Pm_sys_c_ES3 : Constant  Value=Pm_3
  Pm_sys_c_ES4 : Constant  Value=Pm_4
  Pm_sys_c_G1 : Constant  Value=Pmg_1
  Pm_sys_c_G2 : Constant  Value=Pmg_2
  Pm_sys_c_G3 : Constant  Value=Pmg_3
  RI2C_ES{1..4} (4 alike) : RealImagToComplex
  RI2C_G1 : RealImagToComplex
  RI2C_G2 : RealImagToComplex
  RI2C_G3 : RealImagToComplex
  SCvar_c_ES1 : Constant  Value=VSGScale_1
  SCvar_c_ES2 : Constant  Value=VSGScale_2
  SCvar_c_ES3 : Constant  Value=VSGScale_3
  SCvar_c_ES4 : Constant  Value=VSGScale_4
  SCvar_c_G1 : Constant  Value=SGScale_1
  SCvar_c_G2 : Constant  Value=SGScale_2
  SCvar_c_G3 : Constant  Value=SGScale_3
  Shunt7 : spsSeriesRLCBranchLib/Series RLC Branch  LConnTagsString=__new0  RConnTagsString=__new0  BranchType=C  Resistance=1  Inductance=1e-3  SetiL0=off  InitialCurrent=0  Capacitance=1.203440023e-05  Setx0=off  InitialVoltage=0  Measurements=None
  Shunt9 : spsSeriesRLCBranchLib/Series RLC Branch  LConnTagsString=__new0  RConnTagsString=__new0  BranchType=C  Resistance=1  Inductance=1e-3  SetiL0=off  InitialCurrent=0  Capacitance=2.106020041e-05  Setx0=off  InitialVoltage=0  Measurements=None
  Sscale_c_ES1 : Constant  Value=VSGScale_1
  Sscale_c_ES2 : Constant  Value=VSGScale_2
  Sscale_c_ES3 : Constant  Value=VSGScale_3
  Sscale_c_ES4 : Constant  Value=VSGScale_4
  Sscale_c_G1 : Constant  Value=SGScale_1
  Sscale_c_G2 : Constant  Value=SGScale_2
  Sscale_c_G3 : Constant  Value=SGScale_3
  SumDw_ES{1..4} (4 alike) : Sum  Inputs=+-
  SumDw_G1 : Sum  Inputs=+-
  SumDw_G2 : Sum  Inputs=+-
  SumDw_G3 : Sum  Inputs=+-
  SwingSum_ES{1..4} (4 alike) : Sum  Inputs=+--
  SwingSum_G1 : Sum  Inputs=+--
  SwingSum_G2 : Sum  Inputs=+--
  SwingSum_G3 : Sum  Inputs=+--
  V_RI_ES{1..4} (4 alike) : ComplexToRealImag
  V_RI_G1 : ComplexToRealImag
  V_RI_G2 : ComplexToRealImag
  V_RI_G3 : ComplexToRealImag
  ViG_ES1 : Gain  Gain=Vmag_1
  ViG_ES2 : Gain  Gain=Vmag_2
  ViG_ES3 : Gain  Gain=Vmag_3
  ViG_ES4 : Gain  Gain=Vmag_4
  ViG_G1 : Gain  Gain=VemfG_1
  ViG_G2 : Gain  Gain=VemfG_2
  ViG_G3 : Gain  Gain=VemfG_3
  ViIi_ES{1..4} (4 alike) : Product
  ViIi_G1 : Product
  ViIi_G2 : Product
  ViIi_G3 : Product
  Vmeas_ES{1..4} (4 alike) : spsVoltageMeasurementLib/Voltage Measurement  PhasorSimulation=on  OutputType=Complex  PSBequivalent=0
  Vmeas_G1 : spsVoltageMeasurementLib/Voltage Measurement  PhasorSimulation=on  OutputType=Complex  PSBequivalent=0
  Vmeas_G2 : spsVoltageMeasurementLib/Voltage Measurement  PhasorSimulation=on  OutputType=Complex  PSBequivalent=0
  Vmeas_G3 : spsVoltageMeasurementLib/Voltage Measurement  PhasorSimulation=on  OutputType=Complex  PSBequivalent=0
  VrG_ES1 : Gain  Gain=Vmag_1
  VrG_ES2 : Gain  Gain=Vmag_2
  VrG_ES3 : Gain  Gain=Vmag_3
  VrG_ES4 : Gain  Gain=Vmag_4
  VrG_G1 : Gain  Gain=VemfG_1
  VrG_G2 : Gain  Gain=VemfG_2
  VrG_G3 : Gain  Gain=VemfG_3
  VrIr_ES{1..4} (4 alike) : Product
  VrIr_G1 : Product
  VrIr_G2 : Product
  VrIr_G3 : Product
  W_Pe_ES1 : ToWorkspace  VariableName=Pe_ts_1  SaveFormat=Timeseries  SampleTime=-1
      settings: MaxDataPoints=2
  W_Pe_ES2 : ToWorkspace  VariableName=Pe_ts_2  SaveFormat=Timeseries  SampleTime=-1
      settings: MaxDataPoints=2
  W_Pe_ES3 : ToWorkspace  VariableName=Pe_ts_3  SaveFormat=Timeseries  SampleTime=-1
      settings: MaxDataPoints=2
  W_Pe_ES4 : ToWorkspace  VariableName=Pe_ts_4  SaveFormat=Timeseries  SampleTime=-1
      settings: MaxDataPoints=2
  W_Pe_G1 : ToWorkspace  VariableName=Pe_ts_G1  SaveFormat=Timeseries  SampleTime=-1
      settings: MaxDataPoints=2
  W_Pe_G2 : ToWorkspace  VariableName=Pe_ts_G2  SaveFormat=Timeseries  SampleTime=-1
      settings: MaxDataPoints=2
  W_Pe_G3 : ToWorkspace  VariableName=Pe_ts_G3  SaveFormat=Timeseries  SampleTime=-1
      settings: MaxDataPoints=2
  W_delta_ES1 : ToWorkspace  VariableName=delta_ts_1  SaveFormat=Timeseries  SampleTime=-1
      settings: MaxDataPoints=2
  W_delta_ES2 : ToWorkspace  VariableName=delta_ts_2  SaveFormat=Timeseries  SampleTime=-1
      settings: MaxDataPoints=2
  W_delta_ES3 : ToWorkspace  VariableName=delta_ts_3  SaveFormat=Timeseries  SampleTime=-1
      settings: MaxDataPoints=2
  W_delta_ES4 : ToWorkspace  VariableName=delta_ts_4  SaveFormat=Timeseries  SampleTime=-1
      settings: MaxDataPoints=2
  W_delta_G1 : ToWorkspace  VariableName=delta_ts_G1  SaveFormat=Timeseries  SampleTime=-1
      settings: MaxDataPoints=2
  W_delta_G2 : ToWorkspace  VariableName=delta_ts_G2  SaveFormat=Timeseries  SampleTime=-1
      settings: MaxDataPoints=2
  W_delta_G3 : ToWorkspace  VariableName=delta_ts_G3  SaveFormat=Timeseries  SampleTime=-1
      settings: MaxDataPoints=2
  W_omega_ES1 : ToWorkspace  VariableName=omega_ts_1  SaveFormat=Timeseries  SampleTime=-1
      settings: MaxDataPoints=2
  W_omega_ES2 : ToWorkspace  VariableName=omega_ts_2  SaveFormat=Timeseries  SampleTime=-1
      settings: MaxDataPoints=2
  W_omega_ES3 : ToWorkspace  VariableName=omega_ts_3  SaveFormat=Timeseries  SampleTime=-1
      settings: MaxDataPoints=2
  W_omega_ES4 : ToWorkspace  VariableName=omega_ts_4  SaveFormat=Timeseries  SampleTime=-1
      settings: MaxDataPoints=2
  W_omega_G1 : ToWorkspace  VariableName=omega_ts_G1  SaveFormat=Timeseries  SampleTime=-1
      settings: MaxDataPoints=2
  W_omega_G2 : ToWorkspace  VariableName=omega_ts_G2  SaveFormat=Timeseries  SampleTime=-1
      settings: MaxDataPoints=2
  W_omega_G3 : ToWorkspace  VariableName=omega_ts_G3  SaveFormat=Timeseries  SampleTime=-1
      settings: MaxDataPoints=2
  cosD_ES{1..4} (4 alike) : Trigonometry  Operator=cos
  cosD_G1 : Trigonometry  Operator=cos
  cosD_G2 : Trigonometry  Operator=cos
  cosD_G3 : Trigonometry  Operator=cos
  powergui : spspowerguiLib/powergui  Priority=1  SimulationMode=Phasor  SampleTime=50e-6  frequency=50  Iterations=50  frequencyindice=60  Pbase=100e6  ErrMax=1e-4  UnitsV=kV  UnitsW=MW  buscounter=0  FunctionMessages=off  echomessages=off  EnableUseOfTLC=off  CurrentSourceSwitches=off  DisableSnubberDevices=off  DisableRonSwitches=off  DisableVfSwitches=off  DisplayEquations=off  AutomaticDiscreteSolvers=off  SolverType=Tustin/Backward Euler (TBE)  Interpol=off  ExternalGateDelay=off  methode=off  Ts=100  x0status=blocks  SPID=on  SwTol=0  HookPort=off  NonlinearTolerance=1e-4  nMaxIteration=100  ContinueOnMaxIteration=off  RestoreLinks=warning  ResistiveCurrentMeasurement=off  Frange=[0:2:500]  Ylog=off  Xlog=on  ShowGrid=off  save=off  variable=ZData  structure=0  ZoomFFT=off  StartTime=0.0  cycles=1  DisplayStyle=1  fundamental=60  FreqAxis=off  MaxFrequency=1000  frequencyindicesteady=1  RmsSteady=1  display=off
  sinD_ES{1..4} (4 alike) : Trigonometry
  sinD_G1 : Trigonometry
  sinD_G2 : Trigonometry
  sinD_G3 : Trigonometry
  wnG_ES{1..4} (4 alike) : Gain  Gain=wn_const
  wnG_G1 : Gain  Gain=wn_const
  wnG_G2 : Gain  Gain=wn_const
  wnG_G3 : Gain  Gain=wn_const
  wires:
  ITripRe_bus14/1 -> ITripRI2C_bus14/1
  ITripIm_bus14/1 -> ITripRI2C_bus14/2
  ITripRI2C_bus14/1 -> LoadStepTrip_bus14/1
  ITripRe_bus15/1 -> ITripRI2C_bus15/1
  ITripIm_bus15/1 -> ITripRI2C_bus15/2
  ITripRI2C_bus15/1 -> LoadStepTrip_bus15/1
  CCSLoadRe_bus7/1 -> CCSLoadRI2C_bus7/1
  CCSLoadIm_bus7/1 -> CCSLoadRI2C_bus7/2
  CCSLoadRI2C_bus7/1 -> CCSLoad_bus7/1
  CCSLoadRe_bus9/1 -> CCSLoadRI2C_bus9/1
  CCSLoadIm_bus9/1 -> CCSLoadRI2C_bus9/2
  CCSLoadRI2C_bus9/1 -> CCSLoad_bus9/1
  Vmeas_G1/1 -> V_RI_G1/1
  Imeas_G1/1 -> I_RI_G1/1
  V_RI_G1/1 -> VrIr_G1/1
  I_RI_G1/1 -> VrIr_G1/2
  V_RI_G1/2 -> ViIi_G1/1
  I_RI_G1/2 -> ViIi_G1/2
  VrIr_G1/1 -> PSum_G1/1
  ViIi_G1/1 -> PSum_G1/2
  PSum_G1/1 -> Pe_pu_G1/1
  Clock_global/1 -> GE_G1/1, GE_G2/1, GE_G3/1, GE_ES1/1, GE_ES2/1, GE_ES3/1, GE_ES4/1
  Pm_step_t_c_G1/1 -> GE_G1/2
  GE_G1/1 -> Cast_G1/1
  Cast_G1/1 -> PmStepMul_G1/1
  Pm_step_amp_c_G1/1 -> PmStepMul_G1/2
  Pm_sys_c_G1/1 -> PmSrcPU_G1/1
  Sscale_c_G1/1 -> PmSrcPU_G1/2
  PmSrcPU_G1/1 -> PmTotal_G1/1
  PmStepMul_G1/1 -> PmTotal_G1/2
  IntW_G1/1 -> SumDw_G1/1, W_omega_G1/1
  One_G1/1 -> SumDw_G1/2
  SumDw_G1/1 -> Dgain_G1/1, InvR_G1/1, wnG_G1/1
  PmTotal_G1/1 -> PmAfterDroop_G1/1
  InvR_G1/1 -> PmAfterDroop_G1/2
  PmAfterDroop_G1/1 -> SwingSum_G1/1
  Pe_pu_G1/1 -> PeSrcPU_G1/1, W_Pe_G1/1
  Dgain_G1/1 -> SwingSum_G1/3
  SCvar_c_G1/1 -> PeSrcPU_G1/2
  PeSrcPU_G1/1 -> SwingSum_G1/2
  SwingSum_G1/1 -> Mgain_G1/1
  Mgain_G1/1 -> IntW_G1/1
  wnG_G1/1 -> IntD_G1/1
  IntD_G1/1 -> cosD_G1/1, sinD_G1/1, W_delta_G1/1
  cosD_G1/1 -> VrG_G1/1
  sinD_G1/1 -> ViG_G1/1
  VrG_G1/1 -> RI2C_G1/1
  ViG_G1/1 -> RI2C_G1/2
  RI2C_G1/1 -> CVS_G1/1
  Vmeas_G2/1 -> V_RI_G2/1
  Imeas_G2/1 -> I_RI_G2/1
  V_RI_G2/1 -> VrIr_G2/1
  I_RI_G2/1 -> VrIr_G2/2
  V_RI_G2/2 -> ViIi_G2/1
  I_RI_G2/2 -> ViIi_G2/2
  VrIr_G2/1 -> PSum_G2/1
  ViIi_G2/1 -> PSum_G2/2
  PSum_G2/1 -> Pe_pu_G2/1
  Pm_step_t_c_G2/1 -> GE_G2/2
  GE_G2/1 -> Cast_G2/1
  Cast_G2/1 -> PmStepMul_G2/1
  Pm_step_amp_c_G2/1 -> PmStepMul_G2/2
  Pm_sys_c_G2/1 -> PmSrcPU_G2/1
  Sscale_c_G2/1 -> PmSrcPU_G2/2
  PmSrcPU_G2/1 -> PmTotal_G2/1
  PmStepMul_G2/1 -> PmTotal_G2/2
  IntW_G2/1 -> SumDw_G2/1, W_omega_G2/1
  One_G2/1 -> SumDw_G2/2
  SumDw_G2/1 -> Dgain_G2/1, InvR_G2/1, wnG_G2/1
  PmTotal_G2/1 -> PmAfterDroop_G2/1
  InvR_G2/1 -> PmAfterDroop_G2/2
  PmAfterDroop_G2/1 -> SwingSum_G2/1
  Pe_pu_G2/1 -> PeSrcPU_G2/1, W_Pe_G2/1
  Dgain_G2/1 -> SwingSum_G2/3
  SCvar_c_G2/1 -> PeSrcPU_G2/2
  PeSrcPU_G2/1 -> SwingSum_G2/2
  SwingSum_G2/1 -> Mgain_G2/1
  Mgain_G2/1 -> IntW_G2/1
  wnG_G2/1 -> IntD_G2/1
  IntD_G2/1 -> cosD_G2/1, sinD_G2/1, W_delta_G2/1
  cosD_G2/1 -> VrG_G2/1
  sinD_G2/1 -> ViG_G2/1
  VrG_G2/1 -> RI2C_G2/1
  ViG_G2/1 -> RI2C_G2/2
  RI2C_G2/1 -> CVS_G2/1
  Vmeas_G3/1 -> V_RI_G3/1
  Imeas_G3/1 -> I_RI_G3/1
  V_RI_G3/1 -> VrIr_G3/1
  I_RI_G3/1 -> VrIr_G3/2
  V_RI_G3/2 -> ViIi_G3/1
  I_RI_G3/2 -> ViIi_G3/2
  VrIr_G3/1 -> PSum_G3/1
  ViIi_G3/1 -> PSum_G3/2
  PSum_G3/1 -> Pe_pu_G3/1
  Pm_step_t_c_G3/1 -> GE_G3/2
  GE_G3/1 -> Cast_G3/1
  Cast_G3/1 -> PmStepMul_G3/1
  Pm_step_amp_c_G3/1 -> PmStepMul_G3/2
  Pm_sys_c_G3/1 -> PmSrcPU_G3/1
  Sscale_c_G3/1 -> PmSrcPU_G3/2
  PmSrcPU_G3/1 -> PmTotal_G3/1
  PmStepMul_G3/1 -> PmTotal_G3/2
  IntW_G3/1 -> SumDw_G3/1, W_omega_G3/1
  One_G3/1 -> SumDw_G3/2
  SumDw_G3/1 -> Dgain_G3/1, InvR_G3/1, wnG_G3/1
  PmTotal_G3/1 -> PmAfterDroop_G3/1
  InvR_G3/1 -> PmAfterDroop_G3/2
  PmAfterDroop_G3/1 -> SwingSum_G3/1
  Pe_pu_G3/1 -> PeSrcPU_G3/1, W_Pe_G3/1
  Dgain_G3/1 -> SwingSum_G3/3
  SCvar_c_G3/1 -> PeSrcPU_G3/2
  PeSrcPU_G3/1 -> SwingSum_G3/2
  SwingSum_G3/1 -> Mgain_G3/1
  Mgain_G3/1 -> IntW_G3/1
  wnG_G3/1 -> IntD_G3/1
  IntD_G3/1 -> cosD_G3/1, sinD_G3/1, W_delta_G3/1
  cosD_G3/1 -> VrG_G3/1
  sinD_G3/1 -> ViG_G3/1
  VrG_G3/1 -> RI2C_G3/1
  ViG_G3/1 -> RI2C_G3/2
  RI2C_G3/1 -> CVS_G3/1
  Vmeas_ES1/1 -> V_RI_ES1/1
  Imeas_ES1/1 -> I_RI_ES1/1
  V_RI_ES1/1 -> VrIr_ES1/1
  I_RI_ES1/1 -> VrIr_ES1/2
  V_RI_ES1/2 -> ViIi_ES1/1
  I_RI_ES1/2 -> ViIi_ES1/2
  VrIr_ES1/1 -> PSum_ES1/1
  ViIi_ES1/1 -> PSum_ES1/2
  PSum_ES1/1 -> Pe_pu_ES1/1
  Pm_step_t_c_ES1/1 -> GE_ES1/2
  GE_ES1/1 -> Cast_ES1/1
  Cast_ES1/1 -> PmStepMul_ES1/1
  Pm_step_amp_c_ES1/1 -> PmStepMul_ES1/2
  Pm_sys_c_ES1/1 -> PmSrcPU_ES1/1
  Sscale_c_ES1/1 -> PmSrcPU_ES1/2
  PmSrcPU_ES1/1 -> PmTotal_ES1/1
  PmStepMul_ES1/1 -> PmTotal_ES1/2
  IntW_ES1/1 -> SumDw_ES1/1, W_omega_ES1/1
  One_ES1/1 -> SumDw_ES1/2
  SumDw_ES1/1 -> Dgain_ES1/1, wnG_ES1/1
  PmTotal_ES1/1 -> SwingSum_ES1/1
  Pe_pu_ES1/1 -> PeSrcPU_ES1/1, W_Pe_ES1/1
  Dgain_ES1/1 -> SwingSum_ES1/3
  SCvar_c_ES1/1 -> PeSrcPU_ES1/2
  PeSrcPU_ES1/1 -> SwingSum_ES1/2
  SwingSum_ES1/1 -> Mgain_ES1/1
  Mgain_ES1/1 -> IntW_ES1/1
  wnG_ES1/1 -> IntD_ES1/1
  IntD_ES1/1 -> cosD_ES1/1, sinD_ES1/1, W_delta_ES1/1
  cosD_ES1/1 -> VrG_ES1/1
  sinD_ES1/1 -> ViG_ES1/1
  VrG_ES1/1 -> RI2C_ES1/1
  ViG_ES1/1 -> RI2C_ES1/2
  RI2C_ES1/1 -> CVS_ES1/1
  Vmeas_ES2/1 -> V_RI_ES2/1
  Imeas_ES2/1 -> I_RI_ES2/1
  V_RI_ES2/1 -> VrIr_ES2/1
  I_RI_ES2/1 -> VrIr_ES2/2
  V_RI_ES2/2 -> ViIi_ES2/1
  I_RI_ES2/2 -> ViIi_ES2/2
  VrIr_ES2/1 -> PSum_ES2/1
  ViIi_ES2/1 -> PSum_ES2/2
  PSum_ES2/1 -> Pe_pu_ES2/1
  Pm_step_t_c_ES2/1 -> GE_ES2/2
  GE_ES2/1 -> Cast_ES2/1
  Cast_ES2/1 -> PmStepMul_ES2/1
  Pm_step_amp_c_ES2/1 -> PmStepMul_ES2/2
  Pm_sys_c_ES2/1 -> PmSrcPU_ES2/1
  Sscale_c_ES2/1 -> PmSrcPU_ES2/2
  PmSrcPU_ES2/1 -> PmTotal_ES2/1
  PmStepMul_ES2/1 -> PmTotal_ES2/2
  IntW_ES2/1 -> SumDw_ES2/1, W_omega_ES2/1
  One_ES2/1 -> SumDw_ES2/2
  SumDw_ES2/1 -> Dgain_ES2/1, wnG_ES2/1
  PmTotal_ES2/1 -> SwingSum_ES2/1
  Pe_pu_ES2/1 -> PeSrcPU_ES2/1, W_Pe_ES2/1
  Dgain_ES2/1 -> SwingSum_ES2/3
  SCvar_c_ES2/1 -> PeSrcPU_ES2/2
  PeSrcPU_ES2/1 -> SwingSum_ES2/2
  SwingSum_ES2/1 -> Mgain_ES2/1
  Mgain_ES2/1 -> IntW_ES2/1
  wnG_ES2/1 -> IntD_ES2/1
  IntD_ES2/1 -> cosD_ES2/1, sinD_ES2/1, W_delta_ES2/1
  cosD_ES2/1 -> VrG_ES2/1
  sinD_ES2/1 -> ViG_ES2/1
  VrG_ES2/1 -> RI2C_ES2/1
  ViG_ES2/1 -> RI2C_ES2/2
  RI2C_ES2/1 -> CVS_ES2/1
  Vmeas_ES3/1 -> V_RI_ES3/1
  Imeas_ES3/1 -> I_RI_ES3/1
  V_RI_ES3/1 -> VrIr_ES3/1
  I_RI_ES3/1 -> VrIr_ES3/2
  V_RI_ES3/2 -> ViIi_ES3/1
  I_RI_ES3/2 -> ViIi_ES3/2
  VrIr_ES3/1 -> PSum_ES3/1
  ViIi_ES3/1 -> PSum_ES3/2
  PSum_ES3/1 -> Pe_pu_ES3/1
  Pm_step_t_c_ES3/1 -> GE_ES3/2
  GE_ES3/1 -> Cast_ES3/1
  Cast_ES3/1 -> PmStepMul_ES3/1
  Pm_step_amp_c_ES3/1 -> PmStepMul_ES3/2
  Pm_sys_c_ES3/1 -> PmSrcPU_ES3/1
  Sscale_c_ES3/1 -> PmSrcPU_ES3/2
  PmSrcPU_ES3/1 -> PmTotal_ES3/1
  PmStepMul_ES3/1 -> PmTotal_ES3/2
  IntW_ES3/1 -> SumDw_ES3/1, W_omega_ES3/1
  One_ES3/1 -> SumDw_ES3/2
  SumDw_ES3/1 -> Dgain_ES3/1, wnG_ES3/1
  PmTotal_ES3/1 -> SwingSum_ES3/1
  Pe_pu_ES3/1 -> PeSrcPU_ES3/1, W_Pe_ES3/1
  Dgain_ES3/1 -> SwingSum_ES3/3
  SCvar_c_ES3/1 -> PeSrcPU_ES3/2
  PeSrcPU_ES3/1 -> SwingSum_ES3/2
  SwingSum_ES3/1 -> Mgain_ES3/1
  Mgain_ES3/1 -> IntW_ES3/1
  wnG_ES3/1 -> IntD_ES3/1
  IntD_ES3/1 -> cosD_ES3/1, sinD_ES3/1, W_delta_ES3/1
  cosD_ES3/1 -> VrG_ES3/1
  sinD_ES3/1 -> ViG_ES3/1
  VrG_ES3/1 -> RI2C_ES3/1
  ViG_ES3/1 -> RI2C_ES3/2
  RI2C_ES3/1 -> CVS_ES3/1
  Vmeas_ES4/1 -> V_RI_ES4/1
  Imeas_ES4/1 -> I_RI_ES4/1
  V_RI_ES4/1 -> VrIr_ES4/1
  I_RI_ES4/1 -> VrIr_ES4/2
  V_RI_ES4/2 -> ViIi_ES4/1
  I_RI_ES4/2 -> ViIi_ES4/2
  VrIr_ES4/1 -> PSum_ES4/1
  ViIi_ES4/1 -> PSum_ES4/2
  PSum_ES4/1 -> Pe_pu_ES4/1
  Pm_step_t_c_ES4/1 -> GE_ES4/2
  GE_ES4/1 -> Cast_ES4/1
  Cast_ES4/1 -> PmStepMul_ES4/1
  Pm_step_amp_c_ES4/1 -> PmStepMul_ES4/2
  Pm_sys_c_ES4/1 -> PmSrcPU_ES4/1
  Sscale_c_ES4/1 -> PmSrcPU_ES4/2
  PmSrcPU_ES4/1 -> PmTotal_ES4/1
  PmStepMul_ES4/1 -> PmTotal_ES4/2
  IntW_ES4/1 -> SumDw_ES4/1, W_omega_ES4/1
  One_ES4/1 -> SumDw_ES4/2
  SumDw_ES4/1 -> Dgain_ES4/1, wnG_ES4/1
  PmTotal_ES4/1 -> SwingSum_ES4/1
  Pe_pu_ES4/1 -> PeSrcPU_ES4/1, W_Pe_ES4/1
  Dgain_ES4/1 -> SwingSum_ES4/3
  SCvar_c_ES4/1 -> PeSrcPU_ES4/2
  PeSrcPU_ES4/1 -> SwingSum_ES4/2
  SwingSum_ES4/1 -> Mgain_ES4/1
  Mgain_ES4/1 -> IntW_ES4/1
  wnG_ES4/1 -> IntD_ES4/1
  IntD_ES4/1 -> cosD_ES4/1, sinD_ES4/1, W_delta_ES4/1
  cosD_ES4/1 -> VrG_ES4/1
  sinD_ES4/1 -> ViG_ES4/1
  VrG_ES4/1 -> RI2C_ES4/1
  ViG_ES4/1 -> RI2C_ES4/2
  RI2C_ES4/1 -> CVS_ES4/1
  connections:
  L_1_5_Csh_F/RConn1 -- L_1_5_Csh_F_GND/LConn1
  L_1_5_Csh_T/RConn1 -- L_1_5_Csh_T_GND/LConn1
  L_2_6_Csh_F/RConn1 -- L_2_6_Csh_F_GND/LConn1
  L_2_6_Csh_T/RConn1 -- L_2_6_Csh_T_GND/LConn1
  L_3_10_Csh_F/RConn1 -- L_3_10_Csh_F_GND/LConn1
  L_3_10_Csh_T/RConn1 -- L_3_10_Csh_T_GND/LConn1
  L_4_9_Csh_F/RConn1 -- L_4_9_Csh_F_GND/LConn1
  L_4_9_Csh_T/RConn1 -- L_4_9_Csh_T_GND/LConn1
  L_5_6a_Csh_F/RConn1 -- L_5_6a_Csh_F_GND/LConn1
  L_5_6a_Csh_T/RConn1 -- L_5_6a_Csh_T_GND/LConn1
  L_5_6b_Csh_F/RConn1 -- L_5_6b_Csh_F_GND/LConn1
  L_5_6b_Csh_T/RConn1 -- L_5_6b_Csh_T_GND/LConn1
  L_6_7a_Csh_F/RConn1 -- L_6_7a_Csh_F_GND/LConn1
  L_6_7a_Csh_T/RConn1 -- L_6_7a_Csh_T_GND/LConn1
  L_6_7b_Csh_F/RConn1 -- L_6_7b_Csh_F_GND/LConn1
  L_6_7b_Csh_T/RConn1 -- L_6_7b_Csh_T_GND/LConn1
  L_7_8a_Csh_F/RConn1 -- L_7_8a_Csh_F_GND/LConn1
  L_7_8a_Csh_T/RConn1 -- L_7_8a_Csh_T_GND/LConn1
  L_7_8b_Csh_F/RConn1 -- L_7_8b_Csh_F_GND/LConn1
  L_7_8b_Csh_T/RConn1 -- L_7_8b_Csh_T_GND/LConn1
  L_7_8c_Csh_F/RConn1 -- L_7_8c_Csh_F_GND/LConn1
  L_7_8c_Csh_T/RConn1 -- L_7_8c_Csh_T_GND/LConn1
  L_8_9a_Csh_F/RConn1 -- L_8_9a_Csh_F_GND/LConn1
  L_8_9a_Csh_T/RConn1 -- L_8_9a_Csh_T_GND/LConn1
  L_8_9b_Csh_F/RConn1 -- L_8_9b_Csh_F_GND/LConn1
  L_8_9b_Csh_T/RConn1 -- L_8_9b_Csh_T_GND/LConn1
  L_9_10a_Csh_F/RConn1 -- L_9_10a_Csh_F_GND/LConn1
  L_9_10a_Csh_T/RConn1 -- L_9_10a_Csh_T_GND/LConn1
  L_9_10b_Csh_F/RConn1 -- L_9_10b_Csh_F_GND/LConn1
  L_9_10b_Csh_T/RConn1 -- L_9_10b_Csh_T_GND/LConn1
  L_7_12_Csh_F/RConn1 -- L_7_12_Csh_F_GND/LConn1
  L_7_12_Csh_T/RConn1 -- L_7_12_Csh_T_GND/LConn1
  L_8_16_Csh_F/RConn1 -- L_8_16_Csh_F_GND/LConn1
  L_8_16_Csh_T/RConn1 -- L_8_16_Csh_T_GND/LConn1
  L_10_14_Csh_F/RConn1 -- L_10_14_Csh_F_GND/LConn1
  L_10_14_Csh_T/RConn1 -- L_10_14_Csh_T_GND/LConn1
  L_9_15_Csh_F/RConn1 -- L_9_15_Csh_F_GND/LConn1
  L_9_15_Csh_T/RConn1 -- L_9_15_Csh_T_GND/LConn1
  Load7/RConn1 -- GND_Load7/LConn1
  Load9/RConn1 -- GND_Load9/LConn1
  Shunt7/RConn1 -- GND_Shunt7/LConn1
  Shunt9/RConn1 -- GND_Shunt9/LConn1
  LoadStep_bus14/RConn1 -- GND_LoadStep_bus14/LConn1
  LoadStep_bus15/RConn1 -- GND_LoadStep_bus15/LConn1
  LoadStepTrip_bus14/LConn1 -- GND_LoadStepTrip_bus14/LConn1
  LoadStepTrip_bus15/LConn1 -- GND_LoadStepTrip_bus15/LConn1
  CCSLoad_bus7/LConn1 -- GND_CCSLoad_bus7/LConn1
  CCSLoad_bus9/LConn1 -- GND_CCSLoad_bus9/LConn1
  Imeas_G1/LConn1 -- CVS_G1/RConn1 -- Vmeas_G1/LConn1
  Imeas_G1/RConn1 -- Lint_G1/LConn1
  GND_G1/LConn1 -- CVS_G1/LConn1 -- Vmeas_G1/LConn2
  Imeas_G2/LConn1 -- CVS_G2/RConn1 -- Vmeas_G2/LConn1
  Imeas_G2/RConn1 -- Lint_G2/LConn1
  GND_G2/LConn1 -- CVS_G2/LConn1 -- Vmeas_G2/LConn2
  Imeas_G3/LConn1 -- CVS_G3/RConn1 -- Vmeas_G3/LConn1
  Imeas_G3/RConn1 -- Lint_G3/LConn1
  GND_G3/LConn1 -- CVS_G3/LConn1 -- Vmeas_G3/LConn2
  Imeas_ES1/LConn1 -- CVS_ES1/RConn1 -- Vmeas_ES1/LConn1
  Imeas_ES1/RConn1 -- Lint_ES1/LConn1
  GND_ES1/LConn1 -- CVS_ES1/LConn1 -- Vmeas_ES1/LConn2
  Imeas_ES2/LConn1 -- CVS_ES2/RConn1 -- Vmeas_ES2/LConn1
  Imeas_ES2/RConn1 -- Lint_ES2/LConn1
  GND_ES2/LConn1 -- CVS_ES2/LConn1 -- Vmeas_ES2/LConn2
  Imeas_ES3/LConn1 -- CVS_ES3/RConn1 -- Vmeas_ES3/LConn1
  Imeas_ES3/RConn1 -- Lint_ES3/LConn1
  GND_ES3/LConn1 -- CVS_ES3/LConn1 -- Vmeas_ES3/LConn2
  Imeas_ES4/LConn1 -- CVS_ES4/RConn1 -- Vmeas_ES4/LConn1
  Imeas_ES4/RConn1 -- Lint_ES4/LConn1
  GND_ES4/LConn1 -- CVS_ES4/LConn1 -- Vmeas_ES4/LConn2
  PVS_W1/LConn1 -- GND_W1/LConn1
  PVS_W1/RConn1 -- Lwind_W1/LConn1
  PVS_W2/LConn1 -- GND_W2/LConn1
  PVS_W2/RConn1 -- Lwind_W2/LConn1
  L_1_5/LConn1 -- L_1_5_Csh_F/LConn1 -- Lint_G1/RConn1
  L_1_5_Csh_T/LConn1 -- L_5_6a/LConn1 -- L_5_6a_Csh_F/LConn1 -- L_5_6b/LConn1 -- L_1_5/RConn1 -- L_5_6b_Csh_F/LConn1
  L_2_6/LConn1 -- L_2_6_Csh_F/LConn1 -- Lint_G2/RConn1
  L_2_6_Csh_T/LConn1 -- L_5_6a/RConn1 -- L_5_6a_Csh_T/LConn1 -- L_5_6b/RConn1 -- L_5_6b_Csh_T/LConn1 -- L_6_7a/LConn1 -- L_6_7a_Csh_F/LConn1 -- L_6_7b/LConn1 -- L_2_6/RConn1 -- L_6_7b_Csh_F/LConn1
  L_3_10/LConn1 -- L_3_10_Csh_F/LConn1 -- Lint_G3/RConn1
  L_3_10_Csh_T/LConn1 -- L_9_10a/RConn1 -- L_9_10a_Csh_T/LConn1 -- L_9_10b/RConn1 -- L_9_10b_Csh_T/LConn1 -- L_10_14/LConn1 -- L_3_10/RConn1 -- L_10_14_Csh_F/LConn1
  L_4_9/LConn1 -- L_4_9_Csh_F/LConn1 -- Lwind_W1/RConn1
  L_4_9_Csh_T/LConn1 -- L_8_9a/RConn1 -- L_8_9a_Csh_T/LConn1 -- L_8_9b/RConn1 -- L_8_9b_Csh_T/LConn1 -- L_9_10a/LConn1 -- L_9_10a_Csh_F/LConn1 -- L_9_10b/LConn1 -- L_9_10b_Csh_F/LConn1 -- L_9_15/LConn1 -- L_9_15_Csh_F/LConn1 -- Load9/LConn1 -- Shunt9/LConn1 -- L_4_9/RConn1 -- CCSLoad_bus9/RConn1
  L_6_7a_Csh_T/LConn1 -- L_6_7b/RConn1 -- L_6_7b_Csh_T/LConn1 -- L_7_8a/LConn1 -- L_7_8a_Csh_F/LConn1 -- L_7_8b/LConn1 -- L_7_8b_Csh_F/LConn1 -- L_7_8c/LConn1 -- L_7_8c_Csh_F/LConn1 -- L_7_12/LConn1 -- L_7_12_Csh_F/LConn1 -- Load7/LConn1 -- Shunt7/LConn1 -- L_6_7a/RConn1 -- CCSLoad_bus7/RConn1
  L_7_8a_Csh_T/LConn1 -- L_7_8b/RConn1 -- L_7_8b_Csh_T/LConn1 -- L_7_8c/RConn1 -- L_7_8c_Csh_T/LConn1 -- L_8_9a/LConn1 -- L_8_9a_Csh_F/LConn1 -- L_8_9b/LConn1 -- L_8_9b_Csh_F/LConn1 -- L_8_16/LConn1 -- L_8_16_Csh_F/LConn1 -- L_7_8a/RConn1 -- Lwind_W2/RConn1
  L_7_12/RConn1 -- L_7_12_Csh_T/LConn1 -- Lint_ES1/RConn1
  L_8_16/RConn1 -- L_8_16_Csh_T/LConn1 -- Lint_ES2/RConn1
  L_10_14_Csh_T/LConn1 -- LoadStep_bus14/LConn1 -- LoadStepTrip_bus14/RConn1 -- L_10_14/RConn1 -- Lint_ES3/RConn1
  L_9_15_Csh_T/LConn1 -- LoadStep_bus15/LConn1 -- LoadStepTrip_bus15/RConn1 -- L_9_15/RConn1 -- Lint_ES4/RConn1
